simulink subsystem "Sample_Catmull_Rom_Pos"  (R2023b)
settings: Solver=VariableStepAuto  StartTime=0.0  StopTime=10.0  RelTol=1e-3
undefined symbols (not defined in the file): Spline_Num_Samples
settings Model: Creator=FIRSTMentor  LastModifiedBy=FIRSTMentor

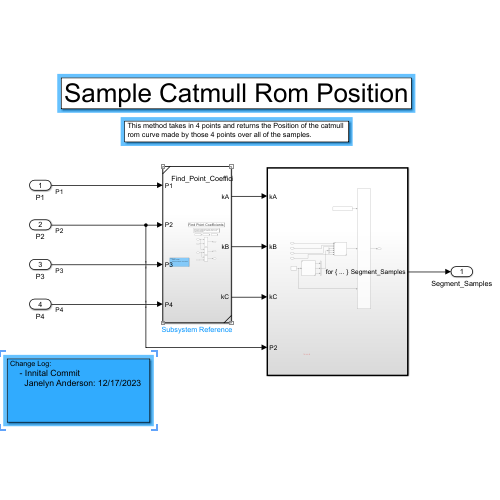
[thumbnail: Simulink's stored preview of the top-level diagram]
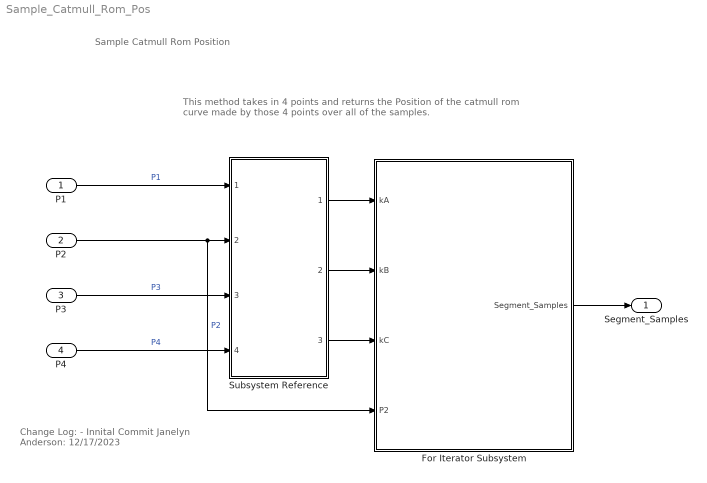
== system Sample_Catmull_Rom_Pos ==
  note: Change Log:
      | - Innital Commit
      | Janelyn Anderson: 12/17/2023
  note: This method takes in 4 points and returns the Position of the catmull rom curve made by those 4 points over all of the samples.
  note: Sample Catmull Rom Position
  P1 : Inport  PortDimensions=[1 2]
  P2 : Inport  Port=2  PortDimensions=[1 2]
  P3 : Inport  Port=3  PortDimensions=[1 2]
  P4 : Inport  Port=4  PortDimensions=[1 2]
  For Iterator Subsystem : Subsystem  TreatAsAtomicUnit=on
  Subsystem Reference : Subsystem  ReferencedSubsystem=Find_Point_Coefficients
  Segment_Samples : Outport
  wires:
  Subsystem Reference/2 -> For Iterator Subsystem/2(kB)
  Subsystem Reference/3 -> For Iterator Subsystem/3(kC)
  P2/1 -> Subsystem Reference/2, For Iterator Subsystem/4(P2)  "P2"
  P4/1 -> Subsystem Reference/4  "P4"
  P1/1 -> Subsystem Reference/1  "P1"
  For Iterator Subsystem/1(Segment_Samples) -> Segment_Samples/1
  P3/1 -> Subsystem Reference/3  "P3"
  Subsystem Reference/1 -> For Iterator Subsystem/1(kA)

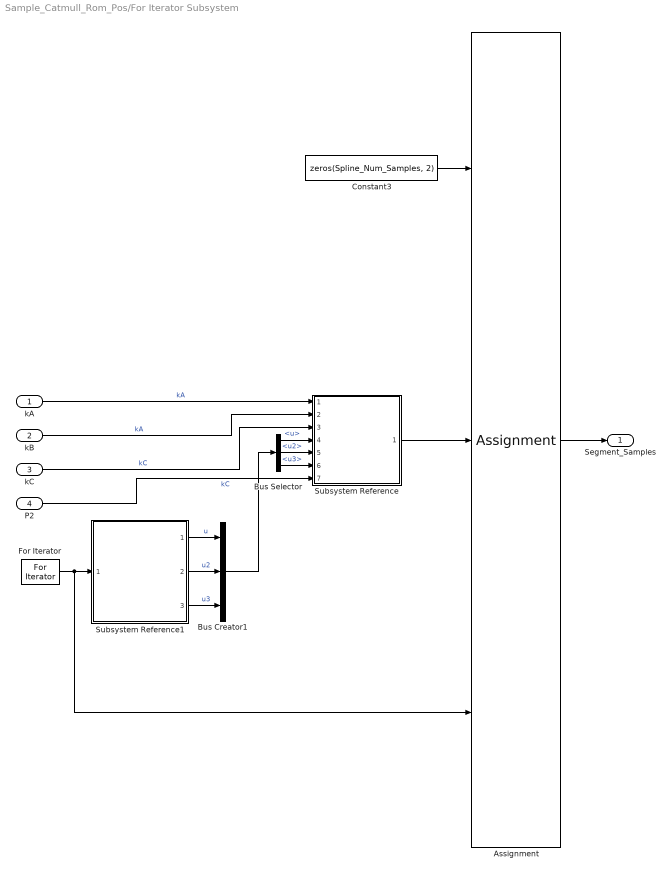
== system Sample_Catmull_Rom_Pos/For Iterator Subsystem ==
  kA : Inport  PortDimensions=[1 2]
  kB : Inport  Port=2  PortDimensions=[1 2]
  kC : Inport  Port=3  PortDimensions=[1 2]
  P2 : Inport  Port=4  PortDimensions=[1 2]
  Assignment : Assignment  NumberOfDimensions=2  DiagnosticForDimensions=Warning  IndexOptions=Index vector (port),Assign all  Indices=1,1  OutputSizes=1,1
  Bus Creator1 : BusCreator  Inputs=3
  Bus Selector : BusSelector  OutputSignals=u,u2,u3
  Constant3 : Constant  Value=zeros(Spline_Num_Samples, 2)
  For Iterator : ForIterator  IterationLimit=Spline_Num_Samples
  Subsystem Reference : Subsystem  ReferencedSubsystem=Find_Catmull_Rom_Pos
  Subsystem Reference1 : Subsystem  ReferencedSubsystem=Find_U_And_Powers
  Segment_Samples : Outport
  wires:
  ? -> ?
  For Iterator/1 -> Subsystem Reference1/1, Assignment/3
  Constant3/1 -> Assignment/1
  Assignment/1 -> Segment_Samples/1
  Bus Creator1/1 -> Bus Selector/1
  Bus Selector/1 -> Subsystem Reference/4  "<u>"
  Bus Selector/3 -> Subsystem Reference/6  "<u3>"
  Bus Selector/2 -> Subsystem Reference/5  "<u2>"
  kA/1 -> Subsystem Reference/1  "kA"
  kB/1 -> Subsystem Reference/2  "kA"
  kC/1 -> Subsystem Reference/3  "kC"
  Subsystem Reference/1 -> Assignment/2
  P2/1 -> Subsystem Reference/7  "kC"
  Subsystem Reference1/2 -> Bus Creator1/2  "u2"
  Subsystem Reference1/1 -> Bus Creator1/1  "u"
  Subsystem Reference1/3 -> Bus Creator1/3  "u3"
